simulink model "TetheredSystem"  (R2016a)
settings: Solver=VariableStepAuto  StartTime=0.0  StopTime=10.0  RelTol=1e-3
settings Model: Creator=cjt79  LastModifiedBy=cjt79
settings GRTTargetCC: GeneratePreprocessorConditionals=Use local settings

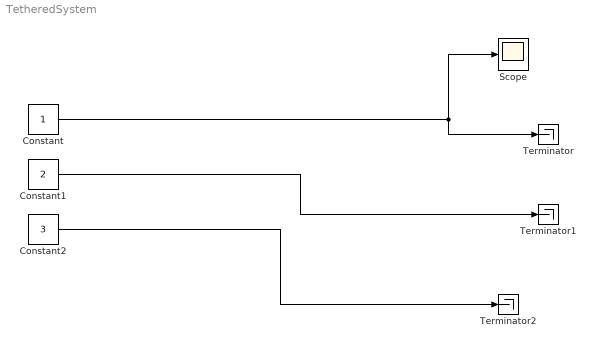
== system TetheredSystem ==
  Constant : Constant
  Constant1 : Constant  Value=2
  Constant2 : Constant  Value=3
  Scope : Scope
  Terminator : Terminator
  Terminator1 : Terminator
  Terminator2 : Terminator
  wires:
  Constant/1 -> Terminator/1, Scope/1
  Constant1/1 -> Terminator1/1
  Constant2/1 -> Terminator2/1
